simulink model "OA_RS"  (R2024b)
settings: Solver=ode3  StartTime=0.0  StopTime=2000  FixedStep=.1  RelTol=1e-3  EnableMultiTasking=on
settings Model: Creator=Ahmed  LastModifiedBy=User
settings SolverCC: AlgebraicLoopSolver=TrustRegion
settings DataIOCC: LimitDataPoints=on  SaveFormat=Array  SignalLoggingSaveFormat=ModelDataLogs  ReturnWorkspaceOutputs=off
settings OptimizationCC: ExpressionDepthLimit=2147483647  LifeSpan=inf
settings DebuggingCC: UnderspecifiedInitializationDetection=Classic  MergeDetectMultiDrivingBlocksExec=none  SolverPrmCheckMsg=warning  UnconnectedInputMsg=warning  UnconnectedOutputMsg=warning  UnconnectedLineMsg=warning  StateNameClashWarn=warning  SFUnexpectedBacktrackingDiag=warning  SFNoUnconditionalDefaultTransitionDiag=warning  SFExecutionAtInitializationDiag=none  ArithmeticOperatorsInVariantConditions=warning
settings HardwareCC: ProdBitPerPointer=32  ProdBitPerSizeT=32  ProdBitPerPtrDiffT=32  ProdLargestAtomicFloat=None  ProdIntDivRoundTo=Undefined  ProdEndianess=Unspecified  ProdWordSize=32  ProdHWDeviceType=32-bit Generic
settings ModelReferenceCC: EnableRefExpFcnMdlSchedulingChecks=on  PropagateSignalLabelsOutOfModel=off
settings SFSimCC: SimUseLocalCustomCode=off  CustomCodeUndefinedFunction=UseInterfaceOnly
settings RTWCC: RTWUseLocalCustomCode=off  GPUComputeCapability=3.5  DLArmComputeVersion=19.05
settings CodeAppCC: StateflowObjectComments=on
settings GRTTargetCC: TargetLangStandard=C89/C90 (ANSI)  CombineOutputUpdateFcns=off  GRTInterface=on
settings ConfigComp: CovMetricSettings=dw  CovSaveCumulativeToWorkspaceVar=on  CovSaveSingleToWorkspaceVar=on  CovExternalEMLEnable=off  CovSFcnEnable=off

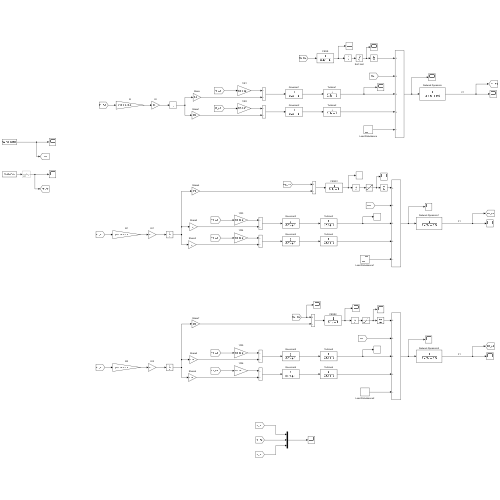
[thumbnail: Simulink's stored preview of the top-level diagram]
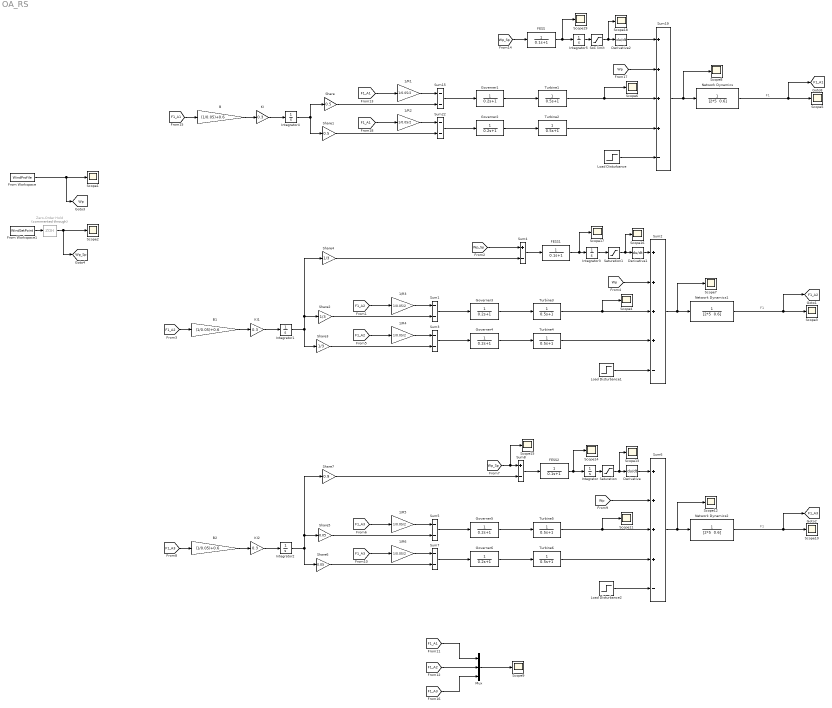
== system OA_RS ==
  note: F1
  note: F1
  note: F1
  1/R{1..6} (6 alike) : Gain  Gain=1/0.05/2
  B : Gain  Gain=(1/0.05)+0.6
  B1 : Gain  Gain=(1/0.05)+0.6
  B2 : Gain  Gain=(1/0.05)+0.6
  Derivative : Derivative
  Derivative1 : Derivative
  Derivative2 : Derivative
  FESS : TransferFcn  Numerator=[0 1]  Denominator="[0.1  1]"
  FESS1 : TransferFcn  Numerator=[0 1]  Denominator="[0.1  1]"
  FESS2 : TransferFcn  Numerator=[0 1]  Denominator="[0.1  1]"
  From Workspace : FromWorkspace  VariableName=WindProfile
  From Workspace1 : FromWorkspace  VariableName=WindSetPoint  SampleTime=-1  Interpolate=off  OutputAfterFinalValue=Holding final value
  Governer{1..6} (6 alike) : TransferFcn  Numerator=[0 1]  Denominator="[0.2  1]"
  Integrator : Integrator  InitialCondition=-9600/15/2
  Integrator1 : Integrator
  Integrator2 : Integrator
  Integrator3 : Integrator  InitialCondition=-9600/15/2
  Integrator4 : Integrator
  Integrator5 : Integrator  InitialCondition=-9600/10/2
  KI : Gain  Gain=0.3
  KI1 : Gain  Gain=0.3
  KI2 : Gain  Gain=0.3
  Load Disturbance : Step  Time=20
  Load Disturbance1 : Step  Time=20
  Load Disturbance2 : Step  Time=20
  Mux : Mux  Inputs=3
  Network Dynamics : TransferFcn  Denominator="[2*5  0.6]"
  Network Dynamics1 : TransferFcn  Denominator="[2*5  0.6]"
  Network Dynamics2 : TransferFcn  Denominator="[2*5  0.6]"
  Saturation : Saturate  UpperLimit=0  LowerLimit=-9600/15
  Saturation1 : Saturate  UpperLimit=0  LowerLimit=-9600/15
  Scope{1..19} (19 alike) : Scope
  Share : Gain  Gain=0.5
  Share1 : Gain  Gain=0.5
  Share2 : Gain  Gain=1/3
  Share3 : Gain  Gain=1/3
  Share4 : Gain  Gain=1/3
  Share5 : Gain  Gain=0.05
  Share6 : Gain  Gain=0.05
  Share7 : Gain  Gain=0.9
  SoC limit : Saturate  UpperLimit=0  LowerLimit=-9600/10
  Sum{1,3,5,7,15,22} (6 alike) : Sum  Inputs=--  InputSameDT=on  SaturateOnIntegerOverflow=on  OutDataTypeStr=Inherit: Same as first input
  Sum19 : Sum  Inputs=++++-  InputSameDT=on  SaturateOnIntegerOverflow=on  OutDataTypeStr=Inherit: Same as first input
  Sum2 : Sum  Inputs=++++-  InputSameDT=on  SaturateOnIntegerOverflow=on  OutDataTypeStr=Inherit: Same as first input
  Sum4 : Sum  Inputs=+-  InputSameDT=on  SaturateOnIntegerOverflow=on  OutDataTypeStr=Inherit: Same as first input
  Sum6 : Sum  Inputs=++++-  InputSameDT=on  SaturateOnIntegerOverflow=on  OutDataTypeStr=Inherit: Same as first input
  Sum8 : Sum  Inputs=+-  InputSameDT=on  SaturateOnIntegerOverflow=on  OutDataTypeStr=Inherit: Same as first input
  Turbine{1..6} (6 alike) : TransferFcn  Numerator=[0 1]  Denominator="[0.5  1]"
  Zero-Order Hold : ZeroOrderHold  Commented=through  SampleTime=.1
  tag scope: F1_A1=global, F1_A2=global, F1_A3=global, Wp=global, Wp_Sp=global
  wires:
  From Workspace/1 -> [Wp], Scope1/1
  From Workspace1/1 -> Zero-Order Hold/1
  B/1 -> KI/1
  1/R1/1 -> Sum15/1
  Governer1/1 -> Turbine1/1
  [F1_A1] -> B/1
  Sum15/1 -> Governer1/1
  KI/1 -> Integrator4/1
  Sum19/1 -> Scope8/1, Network Dynamics/1
  Network Dynamics/1 -> Scope5/1, [F1_A1]
  [F1_A1] -> 1/R1/1
  [F1_A1] -> 1/R2/1
  Sum22/1 -> Governer2/1
  Governer2/1 -> Turbine2/1
  1/R2/1 -> Sum22/1
  Integrator4/1 -> Share1/1, Share/1
  Load Disturbance/1 -> Sum19/5
  Share/1 -> Sum15/2
  Share1/1 -> Sum22/2
  Load Disturbance1/1 -> Sum2/5
  Integrator1/1 -> Share4/1, Share2/1, Share3/1
  1/R4/1 -> Sum3/1
  Governer4/1 -> Turbine4/1
  Sum3/1 -> Governer4/1
  [F1_A2] -> 1/R4/1
  [F1_A2] -> 1/R3/1
  Network Dynamics1/1 -> Scope3/1, [F1_A2]
  Sum2/1 -> Network Dynamics1/1, Scope7/1
  KI1/1 -> Integrator1/1
  Sum1/1 -> Governer3/1
  [F1_A2] -> B1/1
  Sum4/1 -> FESS1/1
  Governer3/1 -> Turbine3/1
  1/R3/1 -> Sum1/1
  B1/1 -> KI1/1
  Share2/1 -> Sum1/2
  Share3/1 -> Sum3/2
  Share4/1 -> Sum4/2
  Mux/1 -> Scope9/1
  [Wp_Sp] -> Sum4/1
  [Wp_Sp] -> FESS/1
  [Wp] -> Sum2/2
  [Wp] -> Sum6/2
  [Wp_Sp] -> Scope15/1, Sum8/1
  Share6/1 -> Sum7/2
  Share5/1 -> Sum5/2
  B2/1 -> KI2/1
  1/R5/1 -> Sum5/1
  Governer5/1 -> Turbine5/1
  Sum8/1 -> FESS2/1
  [F1_A3] -> B2/1
  Sum5/1 -> Governer5/1
  KI2/1 -> Integrator2/1
  Sum6/1 -> Scope12/1, Network Dynamics2/1
  Network Dynamics2/1 -> [F1_A3], Scope10/1
  [F1_A3] -> 1/R5/1
  [F1_A3] -> 1/R6/1
  Sum7/1 -> Governer6/1
  Governer6/1 -> Turbine6/1
  1/R6/1 -> Sum7/1
  Integrator2/1 -> Share6/1, Share5/1, Share7/1
  Load Disturbance2/1 -> Sum6/5
  Integrator/1 -> Saturation/1
  Saturation/1 -> Scope13/1, Derivative/1
  Derivative/1 -> Sum6/1
  FESS2/1 -> Scope14/1, Integrator/1
  Saturation1/1 -> Scope16/1, Derivative1/1
  Integrator3/1 -> Saturation1/1
  FESS1/1 -> Scope17/1, Integrator3/1
  Derivative1/1 -> Sum2/1
  SoC limit/1 -> Scope18/1, Derivative2/1
  FESS/1 -> Integrator5/1, Scope19/1
  Integrator5/1 -> SoC limit/1
  Share7/1 -> Sum8/2
  [F1_A1] -> Mux/1
  [F1_A2] -> Mux/2
  [F1_A3] -> Mux/3
  Turbine3/1 -> Scope4/1, Sum2/3
  Turbine4/1 -> Sum2/4
  Turbine5/1 -> Sum6/3, Scope11/1
  Turbine6/1 -> Sum6/4
  Turbine1/1 -> Sum19/3, Scope6/1
  Turbine2/1 -> Sum19/4
  [Wp] -> Sum19/2
  Derivative2/1 -> Sum19/1
  Zero-Order Hold/1 -> [Wp_Sp], Scope2/1
